simulink model "chap2_1sim"  (Simulink 9.0)
settings: Solver=VariableStepAuto  StartTime=0.0  StopTime=10.0  RelTol=1e-3
settings Model: Creator=Administrator  LastModifiedBy=Administrator
settings DataIOCC: SaveFormat=Dataset
settings OptimizationCC: LifeSpan=auto
settings DebuggingCC: UnderspecifiedInitializationDetection=Simplified  MergeDetectMultiDrivingBlocksExec=error  SFUnexpectedBacktrackingDiag=error  SFNoUnconditionalDefaultTransitionDiag=error  SFExecutionAtInitializationDiag=warning
settings HardwareCC: ProdBitPerPointer=64  ProdBitPerSizeT=64  ProdBitPerPtrDiffT=64  ProdLargestAtomicFloat=Float  ProdIntDivRoundTo=Zero  ProdEndianess=LittleEndian  ProdWordSize=64  ProdHWDeviceType=Intel->x86-64 (Windows64)
settings ModelReferenceCC: PropagateSignalLabelsOutOfModel=on
settings CodeAppCC: StateflowObjectComments=off
settings GRTTargetCC: TargetLangStandard=C99 (ISO)
settings ConfigComp: CovMetricSettings=dwe  CovHtmlReporting=off  CovSaveCumulativeToWorkspaceVar=off  CovSaveSingleToWorkspaceVar=off  CovExternalEMLEnable=on

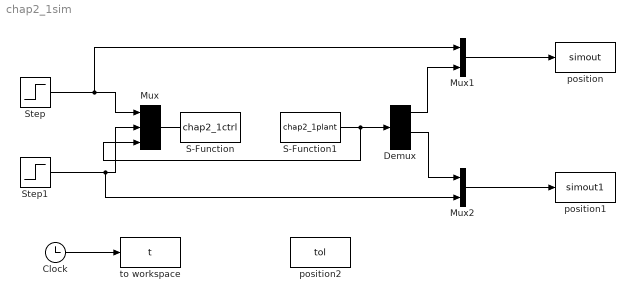
== system chap2_1sim ==
  Clock : Clock
  Demux : Demux
  Mux : Mux  Inputs=3
  Mux1 : Mux  Inputs=2
  Mux2 : Mux  Inputs=2
  S-Function : S-Function  FunctionName=chap2_1ctrl  SFunctionDeploymentMode=off  EnableBusSupport=off
  S-Function1 : S-Function  FunctionName=chap2_1plant  SFunctionDeploymentMode=off  EnableBusSupport=off
  Step : Step  SampleTime=0
  Step1 : Step  SampleTime=0
  position : ToWorkspace  VariableName=simout  SaveFormat=Timeseries  SampleTime=-1
  position1 : ToWorkspace  VariableName=simout1  SaveFormat=Timeseries  SampleTime=-1
  position2 : ToWorkspace  VariableName=tol  SaveFormat=Timeseries  SampleTime=-1
  to workspace : ToWorkspace  VariableName=t  SaveFormat=Timeseries  SampleTime=-1
  wires:
  Step1/1 -> Mux2/2, Mux/2
  Step/1 -> Mux1/1, Mux/1
  S-Function1/1 -> Mux/3, Demux/1
  Demux/1 -> Mux1/2
  Mux1/1 -> position/1
  Mux2/1 -> position1/1
  Demux/3 -> Mux2/1
  Clock/1 -> to workspace/1
  Mux/1 -> ?
